simulink model "FaultDetector_Below20_5Steps"  (R2025a)
settings: Solver=VariableStepAuto  StartTime=0.0  StopTime=10.0  RelTol=1e-3
libraries: simulink x3
settings Model: Creator=mahij  LastModifiedBy=mahij

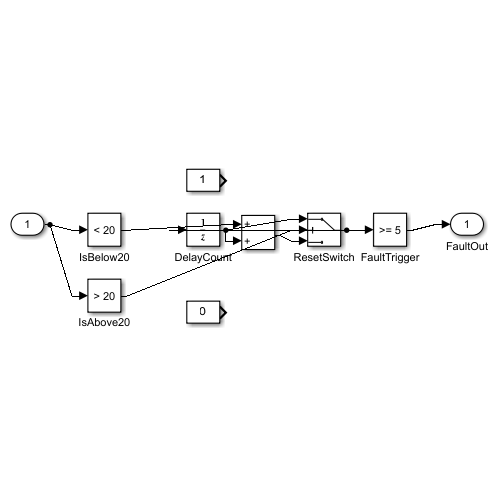
[thumbnail: Simulink's stored preview of the top-level diagram]
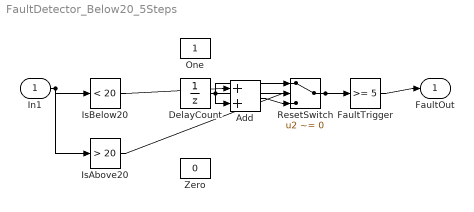
== system FaultDetector_Below20_5Steps ==
  In1 : Inport
  Add : Sum
  DelayCount : UnitDelay  SampleTime=-1  HasFrameUpgradeWarning=on
  FaultTrigger : simulink/Logic and Bit Operations/Compare To Constant  relop=>=  const=5  OutDataTypeStr=boolean
  IsAbove20 : simulink/Logic and Bit Operations/Compare To Constant  relop=>  const=20  OutDataTypeStr=boolean
  IsBelow20 : simulink/Logic and Bit Operations/Compare To Constant  relop=<  const=20  OutDataTypeStr=boolean
  One : Constant
  ResetSwitch : Switch  Criteria=u2 ~= 0  Threshold=0.5  SaturateOnIntegerOverflow=off  InputSameDT=off
  Zero : Constant  Value=0
  FaultOut : Outport
  wires:
  In1/1 -> IsBelow20/1, IsAbove20/1
  IsBelow20/1 -> Add/1
  DelayCount/1 -> Add/2, ResetSwitch/1
  Add/1 -> ResetSwitch/3
  IsAbove20/1 -> ResetSwitch/2
  ResetSwitch/1 -> DelayCount/1, FaultTrigger/1
  FaultTrigger/1 -> FaultOut/1
